simulink model "Mixer"  (R2016a)
settings: Solver=ode2  StartTime=0.0  StopTime=10.0  FixedStep=sample_time  RelTol=1e-3
InitFcn:
  | Parameters_quadrotor
  | Parameters_controllers
undefined symbols (not defined in the file): Kinv, motor_ome_vs_throttle
settings Model: Creator=pela  LastModifiedBy=Mattia
settings DataIOCC: LimitDataPoints=on  SaveFormat=Array
settings HardwareCC: ProdBitPerPointer=32  ProdLargestAtomicInteger=Long  ProdLargestAtomicFloat=Double  ProdIntDivRoundTo=Undefined  ProdWordSize=32  ProdHWDeviceType=ARM Compatible->ARM Cortex
settings ModelReferenceCC: PropagateSignalLabelsOutOfModel=off
settings RTWCC: GenCodeOnly=on  GenerateReport=on  BuildConfiguration=Faster Runs  LaunchReport=on  TargetLang=C++
settings GRTTargetCC: MatFileLogging=off  MultiInstanceERTCode=on  CodeInterfacePackaging=C++ class
settings ConfigComp: CovModelRefEnable=Off

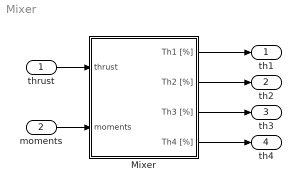
== system Mixer ==
  thrust : Inport
  moments : Inport  Port=2  PortDimensions=3
  Mixer : Subsystem  InitFcn=|
      | %%Parameters definition
      | b = 0.55/2;
      | RPMmax = 3*4.2*710;
      | D = 12*2.54/100;
      | Ct = 0.001;
      | Cq = 0.001;
      | ro = 1.225;
      | 
      | %% From omega squared to forces/torques
      |  A = ro*D^4*diag([Ct b/sqrt(2)*Ct b/sqrt(2)*Ct Cq*D]);
      |  B = [ 1  1  1 1;
      |          1 -1 -1 1;
      |         -1 -1  1 1;
      |         -1  1 -1 1];
      |  C = inv(A*B);       %TM = C * omegasq
  th1 : Outport
  th2 : Outport  Port=2
  th3 : Outport  Port=3
  "th4 " : Outport  Port=4
  wires:
  moments/1 -> Mixer/2(moments)
  Mixer/4(Th4 [%]) -> "th4 "/1
  Mixer/3(Th3 [%]) -> th3/1
  Mixer/2(Th2 [%]) -> th2/1
  Mixer/1(Th1 [%]) -> th1/1
  thrust/1 -> Mixer/1(thrust)

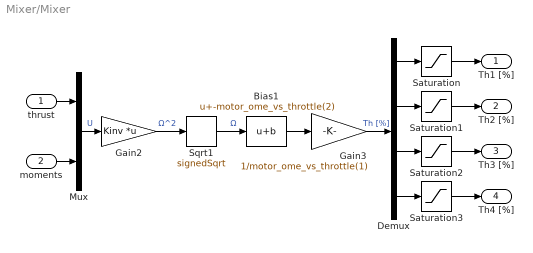
== system Mixer/Mixer ==
  thrust : Inport
  moments : Inport  Port=2  PortDimensions=3
  Bias1 : Bias  Bias=-motor_ome_vs_throttle(2)
  Demux : Demux
  Gain2 : Gain  Gain=Kinv  Multiplication=Matrix(K*u)
  Gain3 : Gain  Gain=1/motor_ome_vs_throttle(1)
  Mux : Mux  Inputs=2
  Saturation{,1..3} (4 alike) : Saturate  UpperLimit=100  LowerLimit=0
  Sqrt1 : Sqrt  Operator=signedSqrt  SaturateOnIntegerOverflow=on
  Th1 [%] : Outport
  Th2 [%] : Outport  Port=2
  Th3 [%] : Outport  Port=3
  Th4 [%] : Outport  Port=4
  wires:
  thrust/1 -> Mux/1
  moments/1 -> Mux/2
  Demux/1 -> Saturation/1
  Saturation/1 -> Th1 [%]/1
  Demux/2 -> Saturation1/1
  Demux/3 -> Saturation2/1
  Demux/4 -> Saturation3/1
  Saturation3/1 -> Th4 [%]/1
  Saturation2/1 -> Th3 [%]/1
  Saturation1/1 -> Th2 [%]/1
  Gain3/1 -> Demux/1  "Th [%]"
  Bias1/1 -> Gain3/1
  Gain2/1 -> Sqrt1/1  "Ω^2"
  Mux/1 -> Gain2/1  "U"
  Sqrt1/1 -> Bias1/1  "Ω"
